simulink model "buck_2016a"  (Simulink 8.7)
settings: Solver=ode23t  StartTime=0.0  StopTime=0.01  MaxStep=1e-7  RelTol=1e-3
libraries: powerlib x19
settings Model: Creator=Asesh Kumar Seth  LastModifiedBy=sayan
settings DataIOCC: LimitDataPoints=off  SaveFormat=Dataset
settings DebuggingCC: UnderspecifiedInitializationDetection=Simplified  MergeDetectMultiDrivingBlocksExec=error
settings HardwareCC: ProdBitPerPointer=64  ProdLargestAtomicFloat=Float  ProdIntDivRoundTo=Zero  ProdEndianess=LittleEndian  ProdWordSize=64  ProdHWDeviceType=Intel->x86-64 (Windows64)
settings ModelReferenceCC: PropagateSignalLabelsOutOfModel=on
settings ConfigComp: CovModelRefEnable=off
settings SimscapeCC: SimscapeNormalizeSystem=off

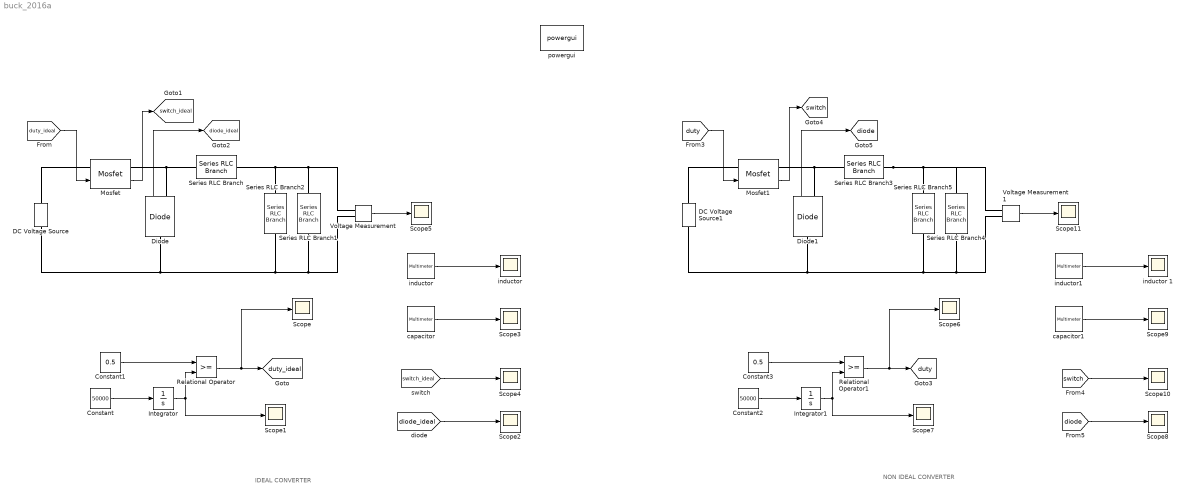
== system buck_2016a ==
  note: NON IDEAL CONVERTER
  note: IDEAL CONVERTER
  Constant : Constant  Value=50000
  Constant1 : Constant  Value=0.5
  Constant2 : Constant  Value=50000
  Constant3 : Constant  Value=0.5
  DC Voltage Source : powerlib/Electrical Sources/DC Voltage Source  Amplitude=110  Measurements=None
  DC Voltage Source1 : powerlib/Electrical Sources/DC Voltage Source  Amplitude=110  Measurements=None
  Diode : powerlib/Power Electronics/Diode  Ron=1e-6  Lon=0  Vf=0  IC=0  UseSnubber=off  Rs=500e6  Cs=250e-9  Measurements=on
  Diode1 : powerlib/Power Electronics/Diode  Ron=1e-6  Lon=0  Vf=0  IC=0  UseSnubber=off  Rs=500e6  Cs=250e-9  Measurements=on
  Integrator : Integrator  UpperSaturationLimit=1  LowerSaturationLimit=0  WrapState=on  WrappedStateUpperValue=1  WrappedStateLowerValue=0
  Integrator1 : Integrator  UpperSaturationLimit=1  LowerSaturationLimit=0  WrapState=on  WrappedStateUpperValue=1  WrappedStateLowerValue=0
  Mosfet : powerlib/Power Electronics/Mosfet  Ron=1e-6  Lon=1e-10  Rd=1e-10  Vfd=0  IC=0  Rs=1e5  Cs=inf  Measurements=on
  Mosfet1 : powerlib/Power Electronics/Mosfet  Ron=100e-3  Lon=1e-10  Rd=1e-10  Vfd=0  IC=0  Rs=1e5  Cs=inf  Measurements=on
  Relational Operator : RelationalOperator  OutDataTypeStr=boolean
  Relational Operator1 : RelationalOperator  OutDataTypeStr=boolean
  Scope{,1..11} (12 alike) : Scope
  Series RLC Branch : powerlib/Elements/Series RLC Branch  LConnTagsString=__new0  RConnTagsString=__new0  BranchType=L  Resistance=1  Inductance=230e-6  SetiL0=off  InitialCurrent=0  Capacitance=1e-6  Setx0=off  InitialVoltage=0  Measurements=Branch voltage and current
  Series RLC Branch1 : powerlib/Elements/Series RLC Branch  LConnTagsString=__new0  RConnTagsString=__new0  BranchType=R  Resistance=11.52  Inductance=1e-3  SetiL0=off  InitialCurrent=0  Capacitance=1e-6  Setx0=off  InitialVoltage=0  Measurements=None
  Series RLC Branch2 : powerlib/Elements/Series RLC Branch  LConnTagsString=__new0  RConnTagsString=__new0  BranchType=C  Resistance=1  Inductance=1e-3  SetiL0=off  InitialCurrent=0  Capacitance=4e-6  Setx0=off  InitialVoltage=0  Measurements=Branch voltage and current
  Series RLC Branch3 : powerlib/Elements/Series RLC Branch  LConnTagsString=__new0  RConnTagsString=__new0  BranchType=RL  Resistance=0.576  Inductance=230e-6  SetiL0=off  InitialCurrent=0  Capacitance=1e-6  Setx0=off  InitialVoltage=0  Measurements=Branch voltage and current
  Series RLC Branch4 : powerlib/Elements/Series RLC Branch  LConnTagsString=__new0  RConnTagsString=__new0  BranchType=R  Resistance=11.52  Inductance=1e-3  SetiL0=off  InitialCurrent=0  Capacitance=1e-6  Setx0=off  InitialVoltage=0  Measurements=None
  Series RLC Branch5 : powerlib/Elements/Series RLC Branch  LConnTagsString=__new0  RConnTagsString=__new0  BranchType=C  Resistance=1  Inductance=1e-3  SetiL0=off  InitialCurrent=0  Capacitance=4e-6  Setx0=off  InitialVoltage=0  Measurements=Branch voltage and current
  Voltage Measurement : powerlib/Measurements/Voltage Measurement  PhasorSimulation=off  OutputType=Complex  PSBequivalent=0
  Voltage Measurement1 : powerlib/Measurements/Voltage Measurement  PhasorSimulation=off  OutputType=Complex  PSBequivalent=0
  capacitor : powerlib/Measurements/Multimeter  PhasorSimulation=off  OutputType=Complex  sel=[2 6]  L=8  Gain=[1 1]  yselected={'Ub: Series RLC Branch2','Ib: Series RLC Branch2'};  PSBOutputType=1  PSBequivalent=0  AxesSetting=[0,0.1,-100,100]  Display=0  SavedBlockNames=-11
  capacitor1 : powerlib/Measurements/Multimeter  PhasorSimulation=off  OutputType=Complex  sel=[2 6]  L=8  Gain=[1 1]  yselected={'Ub: Series RLC Branch2','Ib: Series RLC Branch2'};  PSBOutputType=1  PSBequivalent=0  AxesSetting=[0,0.1,-100,100]  Display=0  SavedBlockNames=-11
  inductor : powerlib/Measurements/Multimeter  PhasorSimulation=off  OutputType=Complex  sel=[1 5]  L=8  Gain=[1 1]  yselected={'Ub: Series RLC Branch','Ib: Series RLC Branch'};  PSBOutputType=1  PSBequivalent=0  AxesSetting=[0,0.1,-100,100]  Display=0  SavedBlockNames=-11
  "inductor " : Scope
  inductor 1 : Scope
  inductor1 : powerlib/Measurements/Multimeter  PhasorSimulation=off  OutputType=Complex  sel=[1 5]  L=8  Gain=[1 1]  yselected={'Ub: Series RLC Branch','Ib: Series RLC Branch'};  PSBOutputType=1  PSBequivalent=0  AxesSetting=[0,0.1,-100,100]  Display=0  SavedBlockNames=-11
  powergui : powerlib/powergui  Priority=1  SimulationMode=Discrete  SampleTime=5e-8  frequency=60  Iterations=50  frequencyindice=0  Pbase=100e6  ErrMax=1e-4  UnitsV=kV  UnitsW=MW  buscounter=0  FunctionMessages=off  echomessages=off  EnableUseOfTLC=off  CurrentSourceSwitches=on  DisableSnubberDevices=off  DisableRonSwitches=off  DisableVfSwitches=off  DisplayEquations=off  SolverType=Tustin/Backward Euler (TBE)  Interpol=off  ExternalGateDelay=off  methode=off  Ts=10  x0status=blocks  SPID=off  SwTol=0  HookPort=off  RestoreLinks=warning  ResistiveCurrentMeasurement=off  Frange=[0:2:500]  Ylog=off  Xlog=on  ShowGrid=off  save=off  variable=ZData  structure=0  ZoomFFT=off  StartTime=0.0  cycles=1  DisplayStyle=1  fundamental=60  FreqAxis=off  MaxFrequency=1000  frequencyindicesteady=1  RmsSteady=1  display=off
  tag scope: diode=global, diode_ideal=global, duty=global, duty_ideal=global, switch=global, switch_ideal=global
  wires:
  Constant/1 -> Integrator/1
  Integrator/1 -> Scope1/1, Relational Operator/2
  Constant1/1 -> Relational Operator/1
  Relational Operator/1 -> Scope/1, [duty_ideal]
  [duty_ideal] -> Mosfet/1
  inductor/1 -> "inductor "/1
  capacitor/1 -> Scope3/1
  Mosfet/1 -> [switch_ideal]
  Diode/1 -> [diode_ideal]
  [switch_ideal] -> Scope4/1
  [diode_ideal] -> Scope2/1
  Voltage Measurement/1 -> Scope5/1
  Constant2/1 -> Integrator1/1
  Integrator1/1 -> Scope7/1, Relational Operator1/2
  Constant3/1 -> Relational Operator1/1
  Relational Operator1/1 -> Scope6/1, [duty]
  [duty] -> Mosfet1/1
  inductor1/1 -> inductor 1/1
  capacitor1/1 -> Scope9/1
  Mosfet1/1 -> [switch]
  Diode1/1 -> [diode]
  [switch] -> Scope10/1
  [diode] -> Scope8/1
  Voltage Measurement1/1 -> Scope11/1
  connections:
  DC Voltage Source/RConn1 -- Mosfet/LConn1
  Series RLC Branch/LConn1 -- Mosfet/RConn1 -- Diode/RConn1
  Series RLC Branch1/LConn1 -- Voltage Measurement/LConn1 -- Series RLC Branch2/LConn1 -- Series RLC Branch/RConn1
  DC Voltage Source/LConn1 -- Series RLC Branch2/RConn1 -- Series RLC Branch1/RConn1 -- Voltage Measurement/LConn2 -- Diode/LConn1
  Diode1/RConn1 -- Series RLC Branch3/LConn1 -- Mosfet1/RConn1
  Series RLC Branch3/RConn1 -- Series RLC Branch5/LConn1 -- Series RLC Branch4/LConn1 -- Voltage Measurement1/LConn1
  Diode1/LConn1 -- DC Voltage Source1/LConn1 -- Series RLC Branch5/RConn1 -- Series RLC Branch4/RConn1 -- Voltage Measurement1/LConn2
  DC Voltage Source1/RConn1 -- Mosfet1/LConn1
